simulink model "pddeffort_red"  (R2020a)
settings: Solver=VariableStepAuto  StartTime=0.0  StopTime=30  RelTol=1e-3
libraries: cstblocks x2
settings Model: Creator=jose  LastModifiedBy=jose

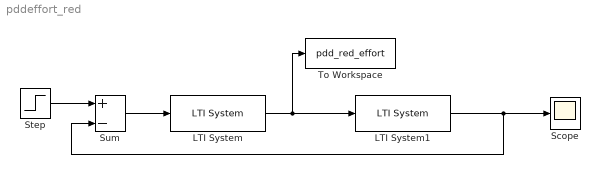
== system pddeffort_red ==
  LTI System : cstblocks/LTI System  sys=Cd_red  IC=[]
  LTI System1 : cstblocks/LTI System  sys=Gd  IC=[]
  Scope : Scope
  Step : Step  Before=1  SampleTime=0
  Sum : Sum  Inputs=+-  InputSameDT=on  SaturateOnIntegerOverflow=on  OutDataTypeStr=Inherit: Same as first input
  To Workspace : ToWorkspace  VariableName=pdd_red_effort  SaveFormat=Timeseries  SampleTime=-1
  wires:
  Step/1 -> Sum/1
  Sum/1 -> LTI System/1
  LTI System/1 -> To Workspace/1, LTI System1/1
  LTI System1/1 -> Scope/1, Sum/2
